simulink model "LimitedSlipDifferential2"  (R2026b)
settings: Solver=VariableStepAuto
libraries: autolibshareddiff x1
settings Model: Creator=The MathWorks, Inc.  LastModifiedBy=The MathWorks, Inc.

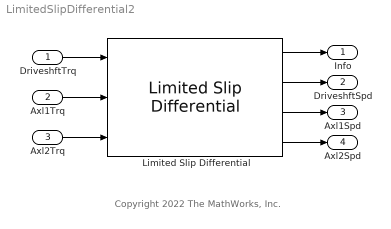
== system LimitedSlipDifferential2 ==
  note: Copyright 2022 The MathWorks, Inc.
  DriveshftTrq : Inport
  Axl1Trq : Inport  Port=2
  Axl2Trq : Inport  Port=3
  Limited Slip Differential : autolibshareddiff/Limited Slip Differential  DiffEffModelPopup=Constant  InterpMethod=Linear point-slope  extTamb=off  shaftSwitchMask=To the left of center-line  Ndiff=4  Jd=.1  bd=1e-3  Jw1=.1  bw1=1e-3  Jw2=.1  bw2=1e-3  omegaw1o=0  omegaw2o=0  eta=1  eta_tbl=PlntDiffrntl2EffTbl  Trq_bpts=PlntDiffrntl2EffTrqBpt  omega_bpts=PlntDiffrntl2EffSpdBpt  Temp_bpts=PlntDiffrntl2EffTempBpt  Tamb=EnvAirTemp  couplingType=Pre-loaded ideal clutch  Ndisks=4  Reff=.20  Fc=500  muc=[.16 0.13 0.115 0.11 0.105 0.1025 0.10125]  dw=[0 10 20 40 60 80 100]  Tdw=PlntDiffrntl2CltchTrqSlipSpdVect  dwT=PlntDiffrntl2CltchSlipSpdVect  TTin=PlntDiffrntl2CltchTrqInTrqVect  Tin=PlntDiffrntl2CltchInTrqVect  tauC=.01  IdealInterpMethod=Linear point-slope  IdealExtrapMethod=Linear  TdwInterpMethod=Flat  TdwExtrapMethod=Clip  TTinInterpMethod=Flat  TTinExtrapMethod=Clip  maxAbsSpd=5e3  aMode=1
      settings: LibrarySourceBlock=autolibdiff/Limited Slip Differential
  Info : Outport
  DriveshftSpd : Outport  Port=2
  Axl1Spd : Outport  Port=3
  Axl2Spd : Outport  Port=4
  wires:
  Limited Slip Differential/1 -> Info/1
  Limited Slip Differential/2 -> DriveshftSpd/1
  Limited Slip Differential/3 -> Axl1Spd/1
  Limited Slip Differential/4 -> Axl2Spd/1
  DriveshftTrq/1 -> Limited Slip Differential/1
  Axl1Trq/1 -> Limited Slip Differential/2
  Axl2Trq/1 -> Limited Slip Differential/3
